simulink model "pv_boost_avg_rload"  (R2020b)
settings: Solver=ode23tb  StartTime=0.0  StopTime=0.1  FixedStep=Ts_Power  RelTol=1e-6  AbsTol=1e-6
libraries: powerlib x17, re_lib x4
Description:
  | Copyright 2008-2019 The MathWorks, Inc.
settings Model: Creator=MathWorks  LastModifiedBy=Balco
settings SolverCC: AutoScaleAbsTol=off  AlgebraicLoopSolver=LineSearch  SolverResetMethod=Robust
settings DataIOCC: LimitDataPoints=on  SaveFormat=Array  SignalLoggingSaveFormat=ModelDataLogs  ReturnWorkspaceOutputs=off
settings OptimizationCC: ExpressionDepthLimit=2147483647  LifeSpan=inf
settings DebuggingCC: UnderspecifiedInitializationDetection=Classic  MergeDetectMultiDrivingBlocksExec=none  FcnCallInpInsideContextMsg=warning  AllowSymbolicDim=off  StateNameClashWarn=warning  SFUnexpectedBacktrackingDiag=warning  SFNoUnconditionalDefaultTransitionDiag=warning  SFExecutionAtInitializationDiag=none  ArithmeticOperatorsInVariantConditions=warning
settings HardwareCC: ProdBitPerPointer=32  ProdBitPerSizeT=32  ProdBitPerPtrDiffT=32  ProdLargestAtomicFloat=None  ProdIntDivRoundTo=Undefined  ProdEndianess=Unspecified  ProdWordSize=32  ProdHWDeviceType=32-bit Generic
settings ModelReferenceCC: PropagateSignalLabelsOutOfModel=off
settings SFSimCC: SimUseLocalCustomCode=off  CustomCodeUndefinedFunction=UseInterfaceOnly
settings RTWCC: RTWUseLocalCustomCode=off
settings CodeAppCC: StateflowObjectComments=on
settings GRTTargetCC: TargetLangStandard=C89/C90 (ANSI)  CombineOutputUpdateFcns=off  GRTInterface=on
settings ConfigComp: CovMetricSettings=dw  CovSaveCumulativeToWorkspaceVar=on  CovSaveSingleToWorkspaceVar=on  CovExternalEMLEnable=off  CovSFcnEnable=off
settings SimscapeCC: SimscapeNormalizeSystem=off

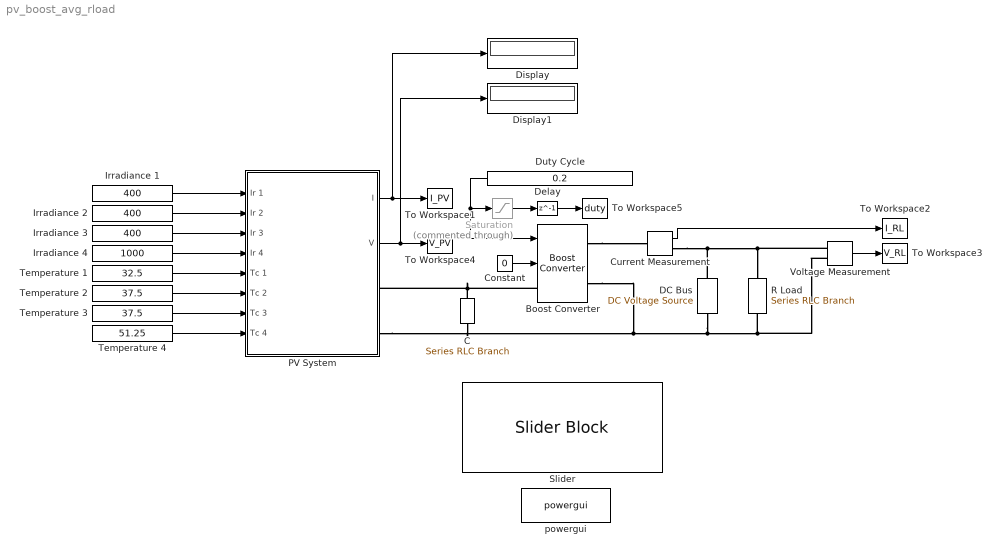
== system pv_boost_avg_rload ==
  Boost Converter : powerlib/Power Electronics/Boost Converter  ModelType=Average model (D-controlled)  Ron=1e-3  Rs=1e6  Cs=inf  Vforward=[0,0]  Ron_Diode=1e-3  Rs_Diode=1e6  Cs_Diode=inf  Vf_Diode=1e-3  Rs_CurrentSource=inf
      settings: SourceProductBaseCode=PS
  C : powerlib/Elements/Series RLC Branch  LConnTagsString=__new0  RConnTagsString=__new0  BranchType=C  Resistance=80  Inductance=1e-3  SetiL0=off  InitialCurrent=0  Capacitance=500e-6  Setx0=on  InitialVoltage=0.0  Measurements=None
  Constant : Constant  Value=0
  Current Measurement : powerlib/Measurements/Current Measurement  PhasorSimulation=off  OutputType=Complex  PSBequivalent=0
  DC Bus : powerlib/Electrical Sources/DC Voltage Source  Amplitude=48  Measurements=None
  Delay : Delay  DelayLength=1  InitialCondition=0
  Display : Display
  Display1 : Display
  Duty Cycle : Constant  Value=0.2
  Irradiance 1 : Constant  Value=400
  Irradiance 2 : Constant  Value=400
  Irradiance 3 : Constant  Value=400
  Irradiance 4 : Constant  Value=1000
  PV System : Subsystem
  R Load : powerlib/Elements/Series RLC Branch  LConnTagsString=__new0  RConnTagsString=__new0  BranchType=R  Resistance=80  Inductance=1e-3  SetiL0=off  InitialCurrent=0  Capacitance=1e-6  Setx0=off  InitialVoltage=0  Measurements=None
  Saturation : Saturate  Commented=through  UpperLimit=1  LowerLimit=0
  Slider : SliderBlock  ScaleMax=1
  Temperature 1 : Constant  Value=32.5
  Temperature 2 : Constant  Value=37.5
  Temperature 3 : Constant  Value=37.5
  Temperature 4 : Constant  Value=51.25
  To Workspace1 : ToWorkspace  VariableName=I_PV  SampleTime=-1
  To Workspace2 : ToWorkspace  VariableName=I_RL  SampleTime=-1
  To Workspace3 : ToWorkspace  VariableName=V_RL  SampleTime=-1
  To Workspace4 : ToWorkspace  VariableName=V_PV  SampleTime=-1
  To Workspace5 : ToWorkspace  VariableName=duty  SampleTime=-1
  Voltage Measurement : powerlib/Measurements/Voltage Measurement  PhasorSimulation=off  OutputType=Complex  PSBequivalent=0
  powergui : powerlib/powergui  Priority=1  SimulationMode=Continuous  SampleTime=1e-9  frequency=60  Iterations=50  frequencyindice=0  Pbase=100e6  ErrMax=1e-4  UnitsV=kV  UnitsW=MW  buscounter=0  FunctionMessages=off  echomessages=off  EnableUseOfTLC=off  CurrentSourceSwitches=on  DisableSnubberDevices=on  DisableRonSwitches=off  DisableVfSwitches=off  DisplayEquations=off  AutomaticDiscreteSolvers=off  SolverType=Tustin/Backward Euler (TBE)  Interpol=off  ExternalGateDelay=off  methode=off  Ts=0  x0status=blocks  SPID=off  SwTol=0  HookPort=off  NonlinearTolerance=0  nMaxIteration=15  ContinueOnMaxIteration=off  RestoreLinks=warning  ResistiveCurrentMeasurement=off  Frange=[0:2:500]  Ylog=off  Xlog=on  ShowGrid=off  save=off  variable=ZData  structure=0  ZoomFFT=on  StartTime=0.0  cycles=1  DisplayStyle=1  fundamental=60  FreqAxis=off  MaxFrequency=1000  frequencyindicesteady=1  RmsSteady=1  display=off
  wires:
  Voltage Measurement/1 -> To Workspace3/1
  Irradiance 1/1 -> PV System/1(Ir 1)
  Temperature 1/1 -> PV System/5(Tc 1)
  Current Measurement/1 -> To Workspace2/1
  Constant/1 -> Boost Converter/2
  Irradiance 2/1 -> PV System/2(Ir 2)
  Irradiance 3/1 -> PV System/3(Ir 3)
  Irradiance 4/1 -> PV System/4(Ir 4)
  Temperature 2/1 -> PV System/6(Tc 2)
  Temperature 3/1 -> PV System/7(Tc 3)
  Temperature 4/1 -> PV System/8(Tc 4)
  Delay/1 -> To Workspace5/1
  Duty Cycle/1 -> Saturation/1, Boost Converter/1
  Saturation/1 -> Delay/1
  PV System/1(I) -> Display/1, To Workspace1/1
  PV System/2(V) -> Display1/1, To Workspace4/1
  connections:
  Voltage Measurement/LConn2 -- PV System/RConn2 -- C/RConn1 -- Boost Converter/RConn2 -- DC Bus/LConn1 -- R Load/RConn1
  Current Measurement/RConn1 -- DC Bus/RConn1 -- Voltage Measurement/LConn1 -- R Load/LConn1
  Boost Converter/RConn1 -- Current Measurement/LConn1
  Boost Converter/LConn1 -- C/LConn1 -- PV System/RConn1

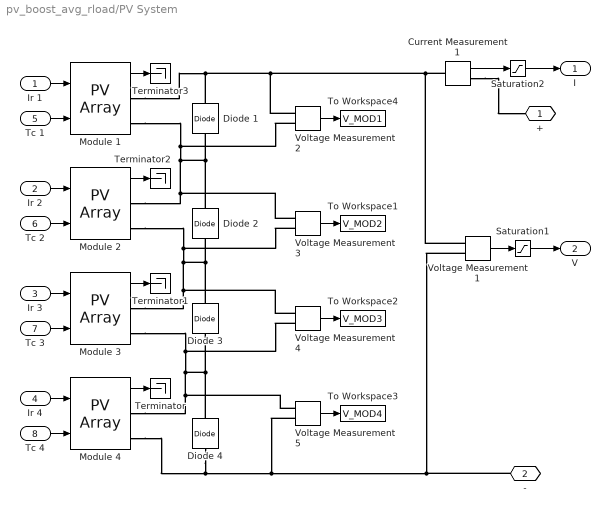
== system pv_boost_avg_rload/PV System ==
  Ir 1 : Inport
  Ir 2 : Inport  Port=2
  Ir 3 : Inport  Port=3
  Ir 4 : Inport  Port=4
  Tc 1 : Inport  Port=5
  Tc 2 : Inport  Port=6
  Tc 3 : Inport  Port=7
  Tc 4 : Inport  Port=8
  Current Measurement1 : powerlib/Measurements/Current Measurement  PhasorSimulation=off  OutputType=Complex  PSBequivalent=0
  Diode {1..4} (4 alike) : powerlib/Power Electronics/Diode  Ron=0.001  Lon=0  Vf=0.8  IC=0  UseSnubber=0  Rs=500  Cs=250e-9  Measurements=off
  Module {1..4} (4 alike) : re_lib/Solar/PV Array  Npar=1  Nser=1  PlotType=array @ 1000 W/m2 & specified temperatures  S_vec="[ 1000  500  100 ]"  Temp_C_vec="[ 45 25  ]"  ModuleName=User-defined  PlotWhenSelected=off  Pm=50.0358  Ncell=12  Voc=32.9/4  Isc=8.21  Vm=26.3/4  Im=7.61  beta_Voc_pc=-0.1230  alpha_Isc_pc=0.0032  beta_Voc=-0.010117  alpha_Isc=0.00026272  IL=8.2568  I0=9.0626e-16  nI=0.72693  Rsh=21.0073  Rs=0.11967  RobustModel=off  RobustCellTemperature=313.3991  BAL=on  Tc=1e-6  Tfilter=5e-8
  Saturation1 : Saturate  UpperLimit=1000  LowerLimit=0
  Saturation2 : Saturate  UpperLimit=1000  LowerLimit=0
  Terminator{,1..3} (4 alike) : Terminator
  To Workspace1 : ToWorkspace  VariableName=V_MOD2  SampleTime=-1
  To Workspace2 : ToWorkspace  VariableName=V_MOD3  SampleTime=-1
  To Workspace3 : ToWorkspace  VariableName=V_MOD4  SampleTime=-1
  To Workspace4 : ToWorkspace  VariableName=V_MOD1  SampleTime=-1
  Voltage Measurement{1..5} (5 alike) : powerlib/Measurements/Voltage Measurement  PhasorSimulation=off  OutputType=Complex  PSBequivalent=0
  + : PMIOPort  Side=Right
  - : PMIOPort  Port=2  Side=Right
  I : Outport
  V : Outport  Port=2
  wires:
  Tc 2/1 -> Module 2/2
  Module 2/1 -> Terminator2/1
  Tc 1/1 -> Module 1/2
  Module 1/1 -> Terminator3/1
  Module 3/1 -> Terminator1/1
  Tc 3/1 -> Module 3/2
  Ir 2/1 -> Module 2/1
  Ir 1/1 -> Module 1/1
  Tc 4/1 -> Module 4/2
  Voltage Measurement1/1 -> Saturation1/1
  Ir 3/1 -> Module 3/1
  Current Measurement1/1 -> Saturation2/1
  Ir 4/1 -> Module 4/1
  Module 4/1 -> Terminator/1
  Voltage Measurement2/1 -> To Workspace4/1
  Voltage Measurement3/1 -> To Workspace1/1
  Voltage Measurement4/1 -> To Workspace2/1
  Voltage Measurement5/1 -> To Workspace3/1
  Saturation1/1 -> V/1
  Saturation2/1 -> I/1
  connections:
  Current Measurement1/RConn1 -- +/RConn1
  Module 1/RConn1 -- Voltage Measurement2/LConn1 -- Current Measurement1/LConn1 -- Voltage Measurement1/LConn1 -- Diode 1/RConn1
  Diode 2/LConn1 -- Diode 3/RConn1 -- Voltage Measurement3/LConn2 -- Module 2/RConn2 -- Voltage Measurement4/LConn1 -- Module 3/RConn1
  Diode 2/RConn1 -- Diode 1/LConn1 -- Voltage Measurement2/LConn2 -- Module 1/RConn2 -- Voltage Measurement3/LConn1 -- Module 2/RConn1
  Voltage Measurement1/LConn2 -- Voltage Measurement5/LConn2 -- Diode 4/LConn1 -- Module 4/RConn2 -- -/RConn1
  Diode 3/LConn1 -- Diode 4/RConn1 -- Voltage Measurement4/LConn2 -- Module 3/RConn2 -- Module 4/RConn1 -- Voltage Measurement5/LConn1
